simulink library "DivisionQuatScalar"  (R2014b)
settings: Solver=ode45  StartTime=0.0  StopTime=10.0  RelTol=1e-3
settings Model: Creator=Hp  LastModifiedBy=Hp

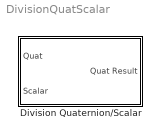
== system DivisionQuatScalar ==
  Division Quaternion/Scalar : Subsystem

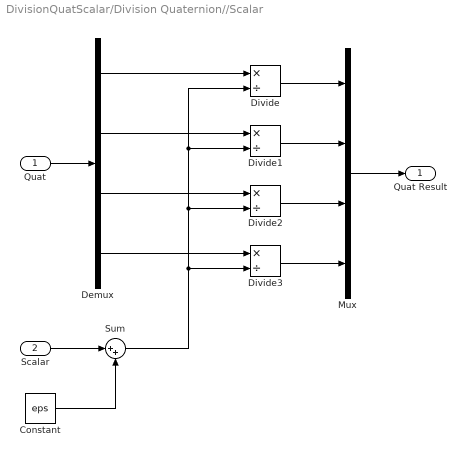
== system DivisionQuatScalar/Division Quaternion//Scalar ==
  Quat : Inport
  Scalar : Inport  Port=2
  Constant : Constant  Value=eps
  Demux : Demux
  Divide{,1..3} (4 alike) : Product  Inputs=*/
  Mux : Mux
  Sum : Sum  Inputs=|++
  Quat Result : Outport
  wires:
  Divide1/1 -> Mux/2
  Quat/1 -> Demux/1
  Divide3/1 -> Mux/4
  Divide/1 -> Mux/1
  Divide2/1 -> Mux/3
  Demux/2 -> Divide1/1
  Constant/1 -> Sum/2
  Demux/3 -> Divide2/1
  Demux/4 -> Divide3/1
  Demux/1 -> Divide/1
  Scalar/1 -> Sum/1
  Mux/1 -> Quat Result/1
  Sum/1 -> Divide2/2, Divide1/2, Divide/2, Divide3/2
